simulink model "untitled1"  (R2023b)
settings: Solver=VariableStepAuto  StartTime=0.0  StopTime=10.0  RelTol=1e-3
model workspace (MAT data in the model file):
  AC_swt_C = Simulink.Signal
  AC_swt_C.DataType = 'auto'
  AC_swt_C.Dimensions = -1
  AC_swt_C.DimensionsMode = 'auto'
  AC_swt_C.Complexity = 'auto'
  AC_swt_C.SampleTime = -1
  AC_swt_C.SamplingMode = 'auto'
  dfsfda.MustResolveToSignalObject = 1
settings Model: Creator=My computer  LastModifiedBy=My computer

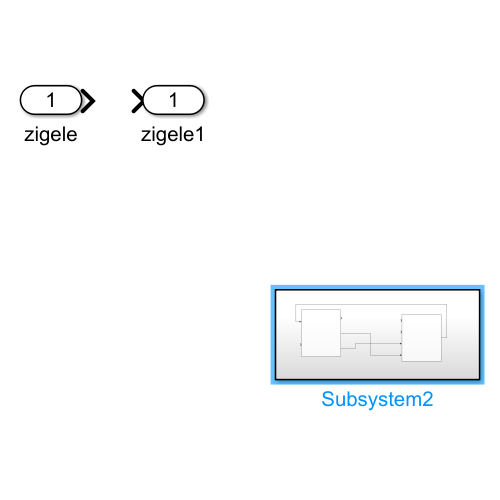
[thumbnail: Simulink's stored preview of the top-level diagram]
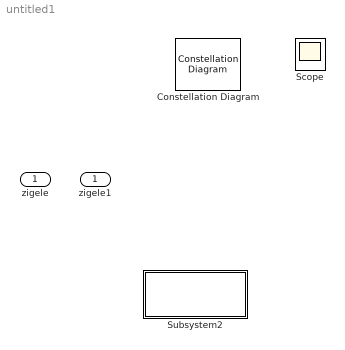
== system untitled1 ==
  zigele : Inport
  Subsystem2 : Subsystem
  zigele1 : Outport
  Constellation Diagram : ConstellationDiagram  IOType=viewer  IsFloating=on  DefaultConfigurationName=comm.scopes.ConstellationDiagramBlockCfg
  Scope : Scope

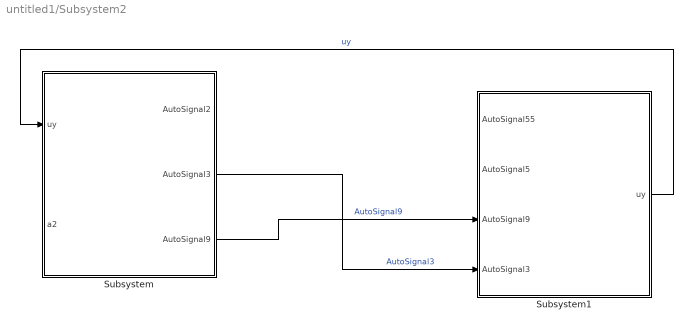
== system untitled1/Subsystem2 ==
  Subsystem : Subsystem
  Subsystem1 : Subsystem
  wires:
  Subsystem/2(AutoSignal3) -> Subsystem1/4(AutoSignal3)  "AutoSignal3"
  Subsystem/3(AutoSignal9) -> Subsystem1/3(AutoSignal9)  "AutoSignal9"
  Subsystem1/1(uy) -> Subsystem/1(uy)  "uy"

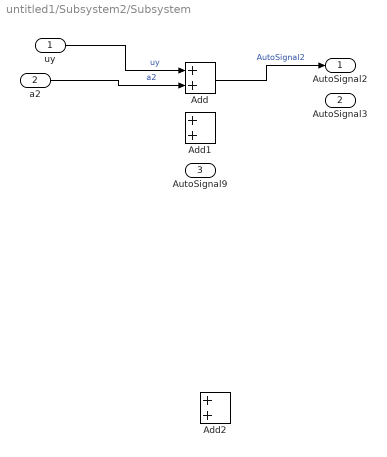
== system untitled1/Subsystem2/Subsystem ==
  uy : Inport
  a2 : Inport  Port=2
  Add : Sum
  Add1 : Sum
  Add2 : Sum
  AutoSignal2 : Outport
  AutoSignal3 : Outport  Port=2
  AutoSignal9 : Outport  Port=3
  wires:
  uy/1 -> Add/1  "uy"
  a2/1 -> Add/2  "a2"
  Add/1 -> AutoSignal2/1  "AutoSignal2"

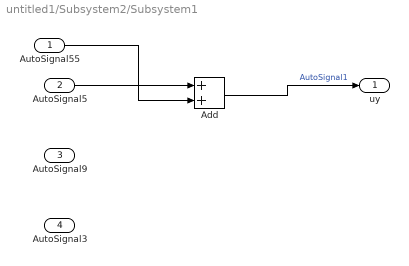
== system untitled1/Subsystem2/Subsystem1 ==
  AutoSignal55 : Inport
  AutoSignal5 : Inport  Port=2
  AutoSignal9 : Inport  Port=3
  AutoSignal3 : Inport  Port=4
  Add : Sum
  uy : Outport
  wires:
  Add/1 -> uy/1  "AutoSignal1"
  AutoSignal55/1 -> Add/2
  AutoSignal5/1 -> Add/1
